simulink model "ejeUR3Simulink"  (R2020b)
settings: Solver=VariableStepAuto  StartTime=0.0  StopTime=15  RelTol=1e-3
libraries: roblocks x2
settings Model: Creator=hunajpu  LastModifiedBy=hunajpu

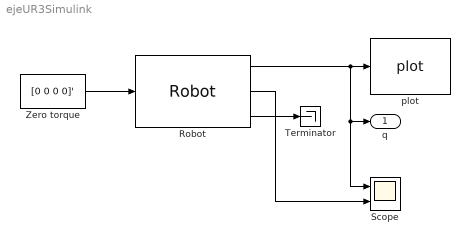
== system ejeUR3Simulink ==
  Robot : roblocks/Arm/Robot  robot=robot.nofriction  q0=[8 0 pi/2 0]
  Scope : Scope  NumInputPorts=2
  Terminator : Terminator
  Zero torque : Constant  Value=[0 0 0 0]'
  plot : roblocks/Arm/plot  robot=robot  fps=25  holdplot=on
  q : Outport
  wires:
  Robot/1 -> plot/1, Scope/1, q/1
  Robot/2 -> Scope/2
  Robot/3 -> Terminator/1
  Zero torque/1 -> Robot/1
